simulink model "pv_boost_avg_rload_thesis_fig"  (R2020b)
settings: Solver=ode23tb  StartTime=0.0  StopTime=0.1  FixedStep=Ts_Power  RelTol=1e-6  AbsTol=1e-6
undefined symbols (not defined in the file): Ion, Lithium
libraries: powerlib x12, re_lib x4, electricdrivelib x1
Description:
  | Copyright 2008-2019 The MathWorks, Inc.
settings Model: Creator=MathWorks  LastModifiedBy=balco
settings SolverCC: AutoScaleAbsTol=off  AlgebraicLoopSolver=LineSearch  SolverResetMethod=Robust
settings DataIOCC: LimitDataPoints=on  SaveFormat=Array  SignalLoggingSaveFormat=ModelDataLogs  ReturnWorkspaceOutputs=off
settings OptimizationCC: ExpressionDepthLimit=2147483647  LifeSpan=inf
settings DebuggingCC: UnderspecifiedInitializationDetection=Classic  MergeDetectMultiDrivingBlocksExec=none  FcnCallInpInsideContextMsg=warning  AllowSymbolicDim=off  StateNameClashWarn=warning  SFUnexpectedBacktrackingDiag=warning  SFNoUnconditionalDefaultTransitionDiag=warning  SFExecutionAtInitializationDiag=none  ArithmeticOperatorsInVariantConditions=warning
settings HardwareCC: ProdBitPerPointer=32  ProdBitPerSizeT=32  ProdBitPerPtrDiffT=32  ProdLargestAtomicFloat=None  ProdIntDivRoundTo=Undefined  ProdEndianess=Unspecified  ProdWordSize=32  ProdHWDeviceType=32-bit Generic
settings ModelReferenceCC: PropagateSignalLabelsOutOfModel=off
settings SFSimCC: SimUseLocalCustomCode=off  CustomCodeUndefinedFunction=UseInterfaceOnly
settings RTWCC: RTWUseLocalCustomCode=off
settings CodeAppCC: StateflowObjectComments=on
settings GRTTargetCC: TargetLangStandard=C89/C90 (ANSI)  CombineOutputUpdateFcns=off  GRTInterface=on
settings ConfigComp: CovMetricSettings=dw  CovSaveCumulativeToWorkspaceVar=on  CovSaveSingleToWorkspaceVar=on  CovExternalEMLEnable=off  CovSFcnEnable=off
settings SimscapeCC: SimscapeNormalizeSystem=off

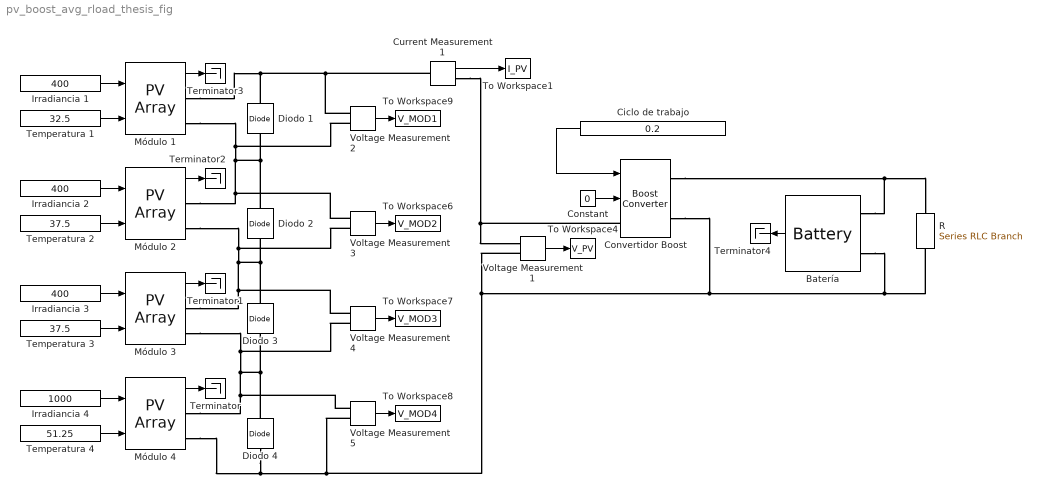
== system pv_boost_avg_rload_thesis_fig ==
  Batería : electricdrivelib/Extra Sources/Battery  BatType=Lithium-Ion  ShowTempParam=off  ThermalPreset=no  ShowAgeParam=off  NomV=7.2  NomQ=5.4  SOC=100  Batt_Tr=30  PresetModel=on  MaxQ=5.4  MinV=5.4  FullV=8.3807  Dis_rate=2.3478  R=0.013333  Normal_OP=4.8835  expZone="[7.7788      0.2653]"  current=[6.5 13 32.5]  Units=Time  Tci=20  NomT=20  T2=-30  MaxQ2=4.8  FullV2=7.1  Normal_OP2=5.655  expZone2="[6.58           1]"  Rca=0.6  ti=2000  Dp=0  Neq0=0  Tsim=1e6  Ta1=25  Qeol=5.4*0.9  Reol=0.013333*1.2  Char_age=[2.3478, 3]  Dis_age=[2.3478, 10]  N1=1500  N2=10500  N3=1000  N4=1400  Ta2=45  N5=950
  Ciclo de trabajo : Constant  Value=0.2
  Constant : Constant  Value=0
  "Convertidor Boost " : powerlib/Power Electronics/Boost Converter  ModelType=Average model (D-controlled)  Ron=1e-3  Rs=1e6  Cs=inf  Vforward=[0,0]  Ron_Diode=1e-3  Rs_Diode=1e6  Cs_Diode=inf  Vf_Diode=1e-3  Rs_CurrentSource=inf
      settings: SourceProductBaseCode=PS
  Current Measurement1 : powerlib/Measurements/Current Measurement  PhasorSimulation=off  OutputType=Complex  PSBequivalent=0
  Diodo {1..4} (4 alike) : powerlib/Power Electronics/Diode  Ron=0.001  Lon=0  Vf=0.8  IC=0  UseSnubber=0  Rs=500  Cs=250e-9  Measurements=off
  Irradiancia 1 : Constant  Value=400
  Irradiancia 2 : Constant  Value=400
  Irradiancia 3 : Constant  Value=400
  Irradiancia 4 : Constant  Value=1000
  Módulo {1..4} (4 alike) : re_lib/Solar/PV Array  Npar=1  Nser=1  PlotType=array @ 1000 W/m2 & specified temperatures  S_vec="[ 1000  500  100 ]"  Temp_C_vec="[ 45 25  ]"  ModuleName=User-defined  PlotWhenSelected=off  Pm=50.0358  Ncell=12  Voc=32.9/4  Isc=8.21  Vm=26.3/4  Im=7.61  beta_Voc_pc=-0.1230  alpha_Isc_pc=0.0032  beta_Voc=-0.010117  alpha_Isc=0.00026272  IL=8.2568  I0=9.0626e-16  nI=0.72693  Rsh=21.0073  Rs=0.11967  RobustModel=off  RobustCellTemperature=313.3991  BAL=on  Tc=1e-6  Tfilter=5e-8
  R : powerlib/Elements/Series RLC Branch  LConnTagsString=__new0  RConnTagsString=__new0  BranchType=R  Resistance=80  Inductance=1e-3  SetiL0=off  InitialCurrent=0  Capacitance=1e-6  Setx0=off  InitialVoltage=0  Measurements=None
  Temperatura 1 : Constant  Value=32.5
  Temperatura 2 : Constant  Value=37.5
  Temperatura 3 : Constant  Value=37.5
  Temperatura 4 : Constant  Value=51.25
  Terminator{,1..4} (5 alike) : Terminator
  To Workspace1 : ToWorkspace  VariableName=I_PV  SampleTime=-1
  To Workspace4 : ToWorkspace  VariableName=V_PV  SampleTime=-1
  To Workspace6 : ToWorkspace  VariableName=V_MOD2  SampleTime=-1
  To Workspace7 : ToWorkspace  VariableName=V_MOD3  SampleTime=-1
  To Workspace8 : ToWorkspace  VariableName=V_MOD4  SampleTime=-1
  To Workspace9 : ToWorkspace  VariableName=V_MOD1  SampleTime=-1
  Voltage Measurement{1..5} (5 alike) : powerlib/Measurements/Voltage Measurement  PhasorSimulation=off  OutputType=Complex  PSBequivalent=0
  wires:
  Constant/1 -> "Convertidor Boost "/2
  Ciclo de trabajo/1 -> "Convertidor Boost "/1
  Voltage Measurement1/1 -> To Workspace4/1
  Voltage Measurement4/1 -> To Workspace7/1
  Voltage Measurement5/1 -> To Workspace8/1
  Voltage Measurement3/1 -> To Workspace6/1
  Voltage Measurement2/1 -> To Workspace9/1
  Módulo 1/1 -> Terminator3/1
  Módulo 3/1 -> Terminator1/1
  Módulo 4/1 -> Terminator/1
  Módulo 2/1 -> Terminator2/1
  Current Measurement1/1 -> To Workspace1/1
  Batería/1 -> Terminator4/1
  Temperatura 4/1 -> Módulo 4/2
  Temperatura 3/1 -> Módulo 3/2
  Temperatura 2/1 -> Módulo 2/2
  Irradiancia 4/1 -> Módulo 4/1
  Irradiancia 3/1 -> Módulo 3/1
  Irradiancia 2/1 -> Módulo 2/1
  Temperatura 1/1 -> Módulo 1/2
  Irradiancia 1/1 -> Módulo 1/1
  connections:
  "Convertidor Boost "/RConn1 -- Batería/LConn1 -- R/LConn1
  Módulo 1/RConn2 -- Diodo 2/RConn1 -- Diodo 1/LConn1 -- Voltage Measurement3/LConn1 -- Módulo 2/RConn1 -- Voltage Measurement2/LConn2
  Diodo 4/RConn1 -- Voltage Measurement4/LConn2 -- Módulo 3/RConn2 -- Módulo 4/RConn1 -- Voltage Measurement5/LConn1 -- Diodo 3/LConn1
  Diodo 3/RConn1 -- Voltage Measurement3/LConn2 -- Módulo 2/RConn2 -- Voltage Measurement4/LConn1 -- Módulo 3/RConn1 -- Diodo 2/LConn1
  Diodo 4/LConn1 -- Módulo 4/RConn2 -- Voltage Measurement1/LConn2 -- "Convertidor Boost "/RConn2 -- Batería/LConn2 -- R/RConn1 -- Voltage Measurement5/LConn2
  "Convertidor Boost "/LConn1 -- Current Measurement1/RConn1 -- Voltage Measurement1/LConn1
  Voltage Measurement2/LConn1 -- Current Measurement1/LConn1 -- Módulo 1/RConn1 -- Diodo 1/RConn1
